simulink model "pendpid"  (Simulink 9.3)
settings: Solver=ode45  StartTime=0.0  StopTime=2  RelTol=1e-3  AbsTol=1e-6
values from neighbouring files (symbols this model uses):
  g = 9.81    [fcn1.m]
undefined symbols (not defined in the file or in its folder): b, i, l, M, m
libraries: simulink x2
settings Model: Creator=nikhil  LastModifiedBy=nikhil
settings OptimizationCC: BlockReduction=off  BooleanDataType=off  LifeSpan=auto
settings DebuggingCC: SaveWithParameterizedLinksMsg=none  SignalResolutionControl=TryResolveAllWithWarning  MultiTaskDSMMsg=warning  MultiTaskCondExecSysMsg=none  FcnCallInpInsideContextMsg=error  SFUnexpectedBacktrackingDiag=error  SFNoUnconditionalDefaultTransitionDiag=error  SFExecutionAtInitializationDiag=warning  ArithmeticOperatorsInVariantConditions=error
settings HardwareCC: ProdBitPerPointer=64  ProdBitPerSizeT=64  ProdBitPerPtrDiffT=64  ProdLargestAtomicFloat=Float  ProdIntDivRoundTo=Zero  ProdEndianess=LittleEndian  ProdWordSize=64  ProdHWDeviceType=Intel->x86-64 (Windows64)  TargetUnknown=on
settings SFSimCC: SimUseLocalCustomCode=on
settings RTWCC: RTWUseLocalCustomCode=on
settings CodeAppCC: StateflowObjectComments=off
settings GRTTargetCC: TargetLangStandard=C99 (ISO)  CombineOutputUpdateFcns=on  GRTInterface=off
settings ConfigComp: CovMetricSettings=dwe  CovHtmlReporting=off  CovSaveCumulativeToWorkspaceVar=off  CovSaveSingleToWorkspaceVar=off  CovExternalEMLEnable=on

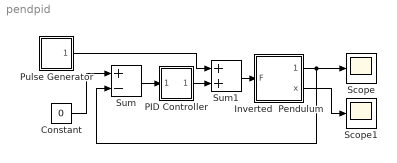
== system pendpid ==
  Constant : Constant  Value=0
  Inverted  Pendulum : Subsystem
  PID Controller : Subsystem  mask(PID Controller){P=100, I=1, D=20}
      mask prompts: P "Proportional:"; I "Integral"; D "Derivative:"
      mask help:
      | Enter expressions for proportional, integral, and derivative terms.
      | P+I/s+Ds
      mask Help: This block implements a PID controller where parameters are entered for the Proportional, Integral and Derivative terms. Unmask this block to see how it works. The derivative term is implemented using a true derivative block.
      mask Display: disp('PID')
  Pulse Generator : Subsystem  mask(Pulse Generator){period=10, duty=.01, amplitude=1000, start=0}
      mask prompts: period "Period (secs):"; duty "Duty cycle (% of period):"; start "Start time:"
      mask help: Pulse Generator
      mask Help: Pulse generator which ensures pulse transitions are hit. Provides a vector of pulses when the height is entered as a vector.  Unmask to see how it works.
      mask Display: plot(0,0,100,100,[95,90,90,75,75,60,60,45,45,30,30,15,15,5],[25,25,75,75,25,25,75,75,25,25,75,75,25,25]);
  Scope : Scope
  Scope1 : Scope
  Sum : Sum  Inputs=+-  SaturateOnIntegerOverflow=on  InputSameDT=on  OutDataTypeStr=Inherit: Same as first input
  Sum1 : Sum  SaturateOnIntegerOverflow=on  InputSameDT=on  OutDataTypeStr=Inherit: Same as first input
  wires:
  Sum/1 -> PID Controller/1(In_1)
  PID Controller/1(Out_1) -> Sum1/2
  Inverted  Pendulum/1(Theta) -> Sum/2, Scope/1
  Constant/1 -> Sum/1
  Pulse Generator/1(out1) -> Sum1/1
  Sum1/1 -> Inverted  Pendulum/1(F)
  Inverted  Pendulum/2(x) -> Scope1/1

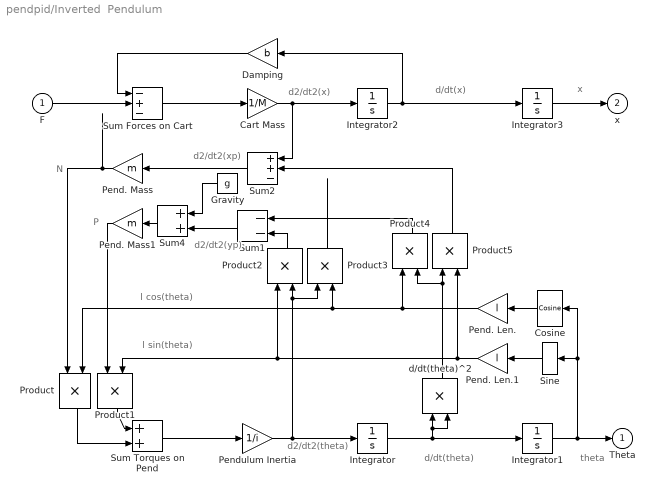
== system pendpid/Inverted  Pendulum ==
  note: d2/dt2(xp)
  note: d2/dt2(yp)
  note: P
  note: N
  note: l sin(theta)
  note: l cos(theta)
  note: x
  note: d/dt(x)
  note: d2/dt2(x)
  note: d2/dt2(theta)
  note: d/dt(theta)
  note: theta
  F : Inport
  Cart Mass : Gain  Gain=1/M  SaturateOnIntegerOverflow=on  OutDataTypeStr=Inherit: Same as input  ParamDataTypeStr=Inherit: Same as input
  Cosine : simulink/Lookup Tables/Cosine  Formula=cos(2*pi*u)  NumDataPoints=(2^5)+1  OutputWordLength=16  InternalRulePriority=Speed
      settings: SourceProductName=Simulink  SourceProductBaseCode=SL
  Damping : Gain  Gain=b  SaturateOnIntegerOverflow=on  OutDataTypeStr=Inherit: Same as input  ParamDataTypeStr=Inherit: Same as input
  Gravity : Constant  Value=g
  Integrator{,1..3} (4 alike) : Integrator
  Pend. Len. : Gain  Gain=l  SaturateOnIntegerOverflow=on  OutDataTypeStr=Inherit: Same as input  ParamDataTypeStr=Inherit: Same as input
  Pend. Len.1 : Gain  Gain=l  SaturateOnIntegerOverflow=on  OutDataTypeStr=Inherit: Same as input  ParamDataTypeStr=Inherit: Same as input
  Pend. Mass : Gain  Gain=m  SaturateOnIntegerOverflow=on  OutDataTypeStr=Inherit: Same as input  ParamDataTypeStr=Inherit: Same as input
  Pend. Mass1 : Gain  Gain=m  SaturateOnIntegerOverflow=on  OutDataTypeStr=Inherit: Same as input  ParamDataTypeStr=Inherit: Same as input
  Pendulum Inertia : Gain  Gain=1/i  SaturateOnIntegerOverflow=on  OutDataTypeStr=Inherit: Same as input  ParamDataTypeStr=Inherit: Same as input
  Product{,1..5} (6 alike) : Product  SaturateOnIntegerOverflow=on  RndMeth=Zero  InputSameDT=on  OutDataTypeStr=Inherit: Same as first input
  Sine : simulink/Lookup Tables/Sine  Formula=sin(2*pi*u)  NumDataPoints=(2^5)+1  OutputWordLength=16  InternalRulePriority=Speed
      settings: SourceProductName=Simulink
  Sum Forces on Cart : Sum  Inputs=-+-  SaturateOnIntegerOverflow=on  InputSameDT=on  OutDataTypeStr=Inherit: Same as first input
  Sum Torques on Pend : Sum  SaturateOnIntegerOverflow=on  InputSameDT=on  OutDataTypeStr=Inherit: Same as first input
  Sum1 : Sum  Inputs=--  SaturateOnIntegerOverflow=on  InputSameDT=on  OutDataTypeStr=Inherit: Same as first input
  Sum2 : Sum  Inputs=++-  SaturateOnIntegerOverflow=on  InputSameDT=on  OutDataTypeStr=Inherit: Same as first input
  Sum4 : Sum  SaturateOnIntegerOverflow=on  InputSameDT=on  OutDataTypeStr=Inherit: Same as first input
  d/dt(theta)^2 : Product  SaturateOnIntegerOverflow=on  RndMeth=Zero  InputSameDT=on  OutDataTypeStr=Inherit: Same as first input
  Theta : Outport  InitialOutput=0
  x : Outport  Port=2  InitialOutput=0
  wires:
  Product2/1 -> Sum1/2
  Product3/1 -> ?
  Product4/1 -> Sum1/1
  Product5/1 -> Sum2/2
  Integrator/1 -> d/dt(theta)^2/2, d/dt(theta)^2/1, Integrator1/1
  Pend. Len.1/1 -> Product5/2, Product2/1, Product1/2
  Pend. Len./1 -> Product4/1, Product3/2, Product/2
  d/dt(theta)^2/1 -> Product4/2, Product5/1
  Pendulum Inertia/1 -> Product2/2, Product3/1, Integrator/1
  Cart Mass/1 -> Sum2/1, Integrator2/1
  Sum2/1 -> Pend. Mass/1
  Sum4/1 -> Pend. Mass1/1
  Sum1/1 -> Sum4/2
  Gravity/1 -> Sum4/1
  Pend. Mass/1 -> Product/1
  Product1/1 -> Sum Torques on Pend/1
  Pend. Mass1/1 -> Product1/1
  Product/1 -> Sum Torques on Pend/2
  Integrator1/1 -> Cosine/1, Sine/1, Theta/1
  Cosine/1 -> Pend. Len./1
  Sine/1 -> Pend. Len.1/1
  F/1 -> Sum Forces on Cart/2
  Damping/1 -> Sum Forces on Cart/1
  Integrator2/1 -> Damping/1, Integrator3/1
  Sum Torques on Pend/1 -> Pendulum Inertia/1
  Sum Forces on Cart/1 -> Cart Mass/1
  Integrator3/1 -> x/1

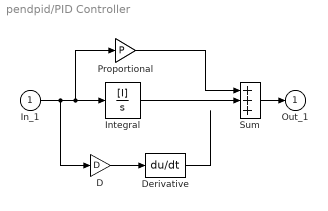
== system pendpid/PID Controller ==
  In_1 : Inport
  D : Gain  Gain=D  SaturateOnIntegerOverflow=on  OutDataTypeStr=Inherit: Same as input  ParamDataTypeStr=Inherit: Same as input
  Derivative : Derivative
  Integral : TransferFcn  Numerator=[I]  Denominator=[1 0]
  Proportional : Gain  Gain=P  SaturateOnIntegerOverflow=on  OutDataTypeStr=Inherit: Same as input  ParamDataTypeStr=Inherit: Same as input
  Sum : Sum  Inputs=+++  SaturateOnIntegerOverflow=on  InputSameDT=on  OutDataTypeStr=Inherit: Same as first input
  Out_1 : Outport  InitialOutput=0
  wires:
  D/1 -> Derivative/1
  Sum/1 -> Out_1/1
  In_1/1 -> D/1, Proportional/1, Integral/1
  Derivative/1 -> ?
  Integral/1 -> Sum/2
  Proportional/1 -> Sum/1

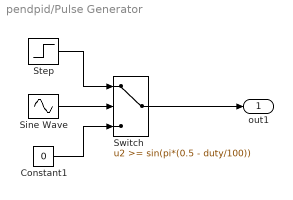
== system pendpid/Pulse Generator ==
  Constant1 : Constant  Value=0
  Sine Wave : Sin  Frequency=2*pi./period  Phase=-2*pi*(start./period + duty/200 - 1/4)
  Step : Step  Time=start  After=amplitude
  Switch : Switch  Threshold=sin(pi*(0.5 - duty/100))  SaturateOnIntegerOverflow=on  InputSameDT=on
  out1 : Outport  InitialOutput=0
  wires:
  Step/1 -> Switch/1
  Constant1/1 -> Switch/3
  Switch/1 -> out1/1
  Sine Wave/1 -> Switch/2
